simulink model "pwm_analysis"  (R2016a)
settings: Solver=ode4  StartTime=0.0  StopTime=Tfinal  FixedStep=Ts  RelTol=1e-3
undefined symbols (not defined in the file or in its folder): Cdc, delta, deltad, fsw, Lload, ma, phase, Rin, Rload, Ts, Vin, wout
libraries: powerlib x21, powerlib_meascontrol x16
settings Model: Creator=ugurm  LastModifiedBy=mesutto
settings DataIOCC: LimitDataPoints=on  SaveFormat=Array
settings DebuggingCC: UnderspecifiedInitializationDetection=Classic  MergeDetectMultiDrivingBlocksExec=none  SolverPrmCheckMsg=warning  StateNameClashWarn=warning
settings HardwareCC: ProdBitPerPointer=32  ProdLargestAtomicFloat=None  ProdIntDivRoundTo=Undefined  ProdEndianess=Unspecified  ProdWordSize=32  ProdHWDeviceType=32-bit Generic
settings ModelReferenceCC: PropagateSignalLabelsOutOfModel=off
settings ConfigComp: CovModelRefEnable=Off

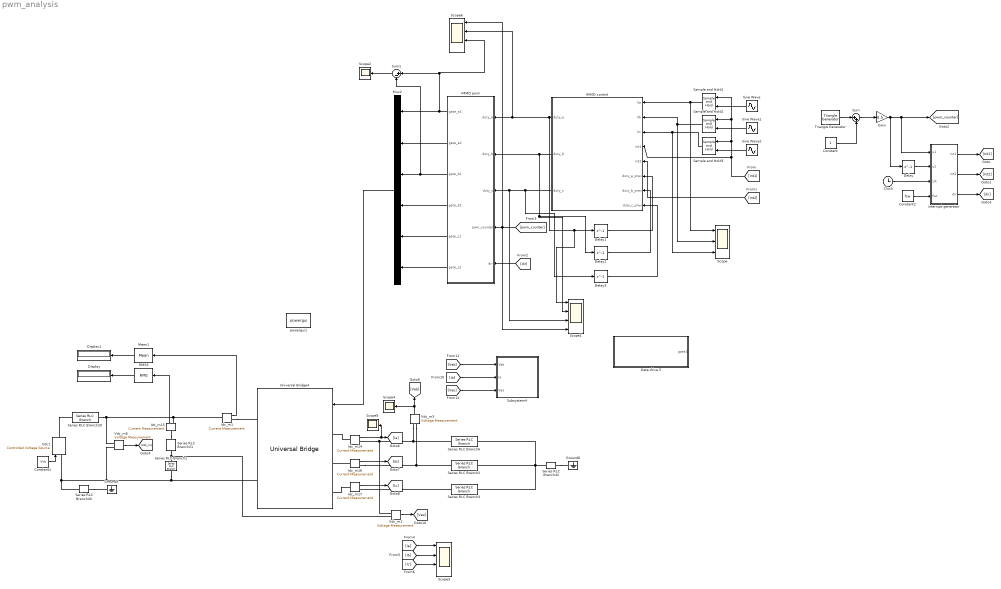
== system pwm_analysis ==
  Clock : Clock
  Constant : Constant
  Constant1 : Constant  Value=Vin
  Constant2 : Constant  Value=fsw
  Delay{,1..3} (4 alike) : Delay  DelayLength=1
  Display : Display
  Display1 : Display
  Gain : Gain  Gain=0.5
  Gate drive 5 : Subsystem
  Ground5 : powerlib/Elements/Ground  LConnTagsString=a
  Ground6 : powerlib/Elements/Ground  LConnTagsString=a
  IMMD control : MATLAB Function  TreatAsAtomicUnit=on
  IMMD pwm : MATLAB Function  TreatAsAtomicUnit=on
  Idc_m{1,14..17} (5 alike) : powerlib/Measurements/Current Measurement  PhasorSimulation=off  OutputType=Complex  PSBequivalent=0
  Mean1 : powerlib_meascontrol/Measurements/Mean  Freq=fout  Vinit=0  Ts=0
  Mux2 : Mux  Inputs=6
  RMS3 : powerlib_meascontrol/Measurements/RMS  TrueRMS=on  Freq=fout  RMSInit=0  Ts=0
  Sample and Hold1 : powerlib_meascontrol/Additional Components/Sample and Hold  ic=0  Ts=0
  Sample and Hold2 : powerlib_meascontrol/Additional Components/Sample and Hold  ic=0  Ts=0
  Sample and Hold3 : powerlib_meascontrol/Additional Components/Sample and Hold  ic=0  Ts=0
  Scope : Scope  NumInputPorts=3
  Scope1 : Scope  NumInputPorts=4
  Scope2 : Scope
  Scope3 : Scope  NumInputPorts=4
  Scope4 : Scope
  Scope5 : Scope
  Scope6 : Scope  NumInputPorts=4
  Series RLC Branch1 : powerlib/Elements/Series RLC Branch  LConnTagsString=__new0  RConnTagsString=__new0  BranchType=C  Resistance=Rload  Inductance=Lload  SetiL0=off  InitialCurrent=0  Capacitance=Cdc*2  Setx0=off  InitialVoltage=0  Measurements=None
  Series RLC Branch2 : powerlib/Elements/Series RLC Branch  LConnTagsString=__new0  RConnTagsString=__new0  BranchType=RL  Resistance=10  Inductance=20e-3  SetiL0=off  InitialCurrent=0  Capacitance=1e-6  Setx0=off  InitialVoltage=0  Measurements=None
  Series RLC Branch20 : powerlib/Elements/Series RLC Branch  LConnTagsString=__new0  RConnTagsString=__new0  BranchType=R  Resistance=Rin  Inductance=Lload  SetiL0=off  InitialCurrent=0  Capacitance=1e-6  Setx0=off  InitialVoltage=0  Measurements=None
  Series RLC Branch21 : powerlib/Elements/Series RLC Branch  LConnTagsString=__new0  RConnTagsString=__new0  BranchType=C  Resistance=Rload  Inductance=Lload  SetiL0=off  InitialCurrent=0  Capacitance=Cdc*2  Setx0=off  InitialVoltage=0  Measurements=None
  Series RLC Branch3 : powerlib/Elements/Series RLC Branch  LConnTagsString=__new0  RConnTagsString=__new0  BranchType=RL  Resistance=10  Inductance=20e-3  SetiL0=off  InitialCurrent=0  Capacitance=1e-6  Setx0=off  InitialVoltage=0  Measurements=None
  Series RLC Branch40 : powerlib/Elements/Series RLC Branch  LConnTagsString=__new0  RConnTagsString=__new0  BranchType=R  Resistance=1e12  Inductance=Lload  SetiL0=off  InitialCurrent=0  Capacitance=1e-6  Setx0=off  InitialVoltage=0  Measurements=None
  Series RLC Branch42 : powerlib/Elements/Series RLC Branch  LConnTagsString=__new0  RConnTagsString=__new0  BranchType=R  Resistance=1e12  Inductance=Lload  SetiL0=off  InitialCurrent=0  Capacitance=1e-6  Setx0=off  InitialVoltage=0  Measurements=None
  Series RLC Branch6 : powerlib/Elements/Series RLC Branch  LConnTagsString=__new0  RConnTagsString=__new0  BranchType=RL  Resistance=10  Inductance=20e-3  SetiL0=off  InitialCurrent=0  Capacitance=1e-6  Setx0=off  InitialVoltage=0  Measurements=None
  Sine Wave : Sin  Amplitude=0.9  Frequency=50*2*pi  SampleTime=0
  Sine Wave1 : Sin  Amplitude=0.9  Frequency=50*2*pi  Phase=2*pi/3  SampleTime=0
  Sine Wave2 : Sin  Amplitude=0.9  Frequency=50*2*pi  Phase=4*pi/3  SampleTime=0
  Subsystem4 : Subsystem
  Sum : Sum  Inputs=|++
  Sum1 : Sum  Inputs=|+-
  Triangle Generator : powerlib_meascontrol/Pulse & Signal Generators/Triangle Generator  Freq=fsw  Phase=0  Ts=0
  Universal Bridge4 : powerlib/Power Electronics/Universal Bridge  Arms=3  SnubberResistance=1e5  SnubberCapacitance=inf  Device=IGBT / Diodes  Ron=1e-6  Lon=0  ForwardVoltages="[  0  0  ]"  ForwardVoltage=0  GTOparameters=[ 10e-6 , 20e-6 ]  IGBTparameters=[0,0]  Measurements=None  Measurements_2=None  converterType=Rectifier
  Vdc1 : powerlib/Electrical Sources/Controlled Voltage Source  Initialize=off  Source_Type=DC  Amplitude=200  Phase=0  Frequency=0  Measurements=None
  Vdc_m1 : powerlib/Measurements/Voltage Measurement  PhasorSimulation=off  OutputType=Complex  PSBequivalent=0
  Vdc_m5 : powerlib/Measurements/Voltage Measurement  PhasorSimulation=off  OutputType=Complex  PSBequivalent=0
  Vdc_m6 : powerlib/Measurements/Voltage Measurement  PhasorSimulation=off  OutputType=Complex  PSBequivalent=0
  interrupt generator : MATLAB Function  TreatAsAtomicUnit=on
  powergui1 : powerlib/powergui  Priority=1  SimulationMode=Discrete  SolverType=Tustin  SampleTime=Ts  frequency=60  SPID=off  DisableSnubberDevices=off  DisableRonSwitches=off  DisableVfSwitches=off  SwTol=0  DisplayEquations=off  Interpol=off  ExternalGateDelay=off  methode=off  Ts=0  FunctionMessages=off  echomessages=off  HookPort=off  EnableUseOfTLC=off  x0status=blocks  frequencyindice=0  Pbase=100e6  ErrMax=1e-4  Iterations=50  UnitsV=kV  UnitsW=MW  buscounter=0  RestoreLinks=warning  ResistiveCurrentMeasurement=off  Frange=[0:2:500]  Ylog=off  Xlog=on  ShowGrid=off  save=off  variable=ZData  structure=ScopeData5  ZoomFFT=off  StartTime=0.02  cycles=2  DisplayStyle=1  fundamental=50  FreqAxis=off  MaxFrequency=50000  frequencyindicesteady=1  RmsSteady=1  display=off
  wires:
  Constant1/1 -> Vdc1/1
  Idc_m15/1 -> RMS3/1
  Vdc_m6/1 -> [Vdc_m]
  RMS3/1 -> Display/1
  Idc_m1/1 -> Mean1/1
  Mean1/1 -> Display1/1
  Triangle Generator/1 -> Sum/1
  Constant/1 -> Sum/2
  Sum/1 -> Gain/1
  Gain/1 -> [pwm_counter], interrupt generator/1(u1), Delay/1
  Delay/1 -> interrupt generator/2(u2)
  Clock/1 -> interrupt generator/3(clk)
  Constant2/1 -> interrupt generator/4(fsw)
  Idc_m14/1 -> Scope5/1, [Ia]
  IMMD pwm/1(gate_a1) -> Scope6/3, Sum1/1, Mux2/1
  IMMD pwm/2(gate_a2) -> Mux2/2
  IMMD pwm/3(gate_b1) -> Sum1/2, Mux2/3
  IMMD pwm/4(gate_b2) -> Mux2/4
  IMMD pwm/5(gate_c1) -> Mux2/5
  IMMD pwm/6(gate_c2) -> Mux2/6
  Sample and Hold3/1 -> Scope/3, IMMD control/3(Vc)
  Sample and Hold2/1 -> Scope/2, IMMD control/2(Vb)
  Sample and Hold1/1 -> Scope/1, IMMD control/1(Va)
  interrupt generator/1(int1) -> [Int1]
  Mux2/1 -> Universal Bridge4/1
  interrupt generator/2(int2) -> [Int2]
  [dir] -> IMMD pwm/5(dir)
  interrupt generator/3(dir) -> [dir]
  [pwm_counter] -> Scope1/4, Scope6/1, IMMD pwm/4(pwm_counter)
  IMMD control/2(duty_b) -> Scope1/2, Delay2/1, IMMD pwm/2(duty_b)
  IMMD control/1(duty_a) -> Scope6/2, IMMD pwm/1(duty_a), Scope1/1, Delay1/1
  [Ia] -> Subsystem4/2(Ia)
  Idc_m16/1 -> [Ib]
  Idc_m17/1 -> [Ic]
  [Vab] -> Subsystem4/1(Vab)
  [Vao] -> Subsystem4/3(Vao)
  Vdc_m5/1 -> [Vab], Scope4/1
  Vdc_m1/1 -> [Vao]
  [Int2] -> IMMD control/5(int2)
  Sine Wave/1 -> Sample and Hold1/1
  Sine Wave1/1 -> Sample and Hold2/1
  Sine Wave2/1 -> Sample and Hold3/1
  [Int1] -> Sample and Hold3/2, Sample and Hold2/2, Sample and Hold1/2, IMMD control/4(int1)
  Delay1/1 -> IMMD control/6(duty_a_prev)
  Delay2/1 -> IMMD control/7(duty_b_prev)
  Delay3/1 -> IMMD control/8(duty_c_prev)
  IMMD control/3(duty_c) -> Delay3/1, Scope1/3, IMMD pwm/3(duty_c)
  Sum1/1 -> Scope2/1
  [Ia] -> Scope3/1
  [Ib] -> Scope3/2
  [Ic] -> Scope3/3
  connections:
  Vdc_m5/LConn1 -- Idc_m14/RConn1 -- Vdc_m1/LConn1 -- Series RLC Branch6/LConn1
  Universal Bridge4/RConn2 -- Vdc_m6/LConn2 -- Vdc1/LConn1 -- Series RLC Branch40/LConn1 -- Series RLC Branch1/RConn1
  Series RLC Branch42/RConn1 -- Ground6/LConn1
  Series RLC Branch40/RConn1 -- Ground5/LConn1
  Idc_m14/LConn1 -- Universal Bridge4/LConn1
  Idc_m15/LConn1 -- Series RLC Branch21/LConn1
  Vdc1/RConn1 -- Series RLC Branch20/LConn1
  Series RLC Branch42/LConn1 -- Series RLC Branch2/RConn1 -- Series RLC Branch3/RConn1 -- Series RLC Branch6/RConn1
  Idc_m16/LConn1 -- Universal Bridge4/LConn2
  Idc_m17/LConn1 -- Universal Bridge4/LConn3
  Series RLC Branch3/LConn1 -- Idc_m17/RConn1
  Idc_m16/RConn1 -- Series RLC Branch2/LConn1 -- Vdc_m5/LConn2
  Idc_m1/RConn1 -- Universal Bridge4/RConn1
  Idc_m1/LConn1 -- Series RLC Branch20/RConn1 -- Vdc_m6/LConn1 -- Idc_m15/RConn1
  Series RLC Branch1/LConn1 -- Vdc_m1/LConn2 -- Series RLC Branch21/RConn1

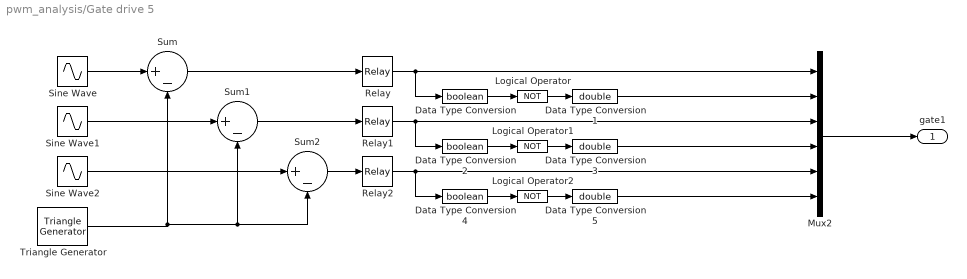
== system pwm_analysis/Gate drive 5 ==
  Data Type Conversion : DataTypeConversion  OutDataTypeStr=boolean
  Data Type Conversion1 : DataTypeConversion  OutDataTypeStr=double
  Data Type Conversion2 : DataTypeConversion  OutDataTypeStr=boolean
  Data Type Conversion3 : DataTypeConversion  OutDataTypeStr=double
  Data Type Conversion4 : DataTypeConversion  OutDataTypeStr=boolean
  Data Type Conversion5 : DataTypeConversion  OutDataTypeStr=double
  Logical Operator : Logic  Operator=NOT  AllPortsSameDT=off  OutDataTypeStr=boolean
  Logical Operator1 : Logic  Operator=NOT  AllPortsSameDT=off  OutDataTypeStr=boolean
  Logical Operator2 : Logic  Operator=NOT  AllPortsSameDT=off  OutDataTypeStr=boolean
  Mux2 : Mux  Inputs=6
  Relay : Relay
  Relay1 : Relay
  Relay2 : Relay
  Sine Wave : Sin  Amplitude=ma  Frequency=wout  Phase=delta  SampleTime=0
  Sine Wave1 : Sin  Amplitude=ma  Frequency=wout  Phase=-2*pi/3+delta  SampleTime=0
  Sine Wave2 : Sin  Amplitude=ma  Frequency=wout  Phase=2*pi/3+delta  SampleTime=0
  Sum : Sum  Inputs=|+-
  Sum1 : Sum  Inputs=|+-
  Sum2 : Sum  Inputs=|+-
  Triangle Generator : powerlib_meascontrol/Pulse & Signal Generators/Triangle Generator  Freq=fsw  Phase=phase(1)  Ts=Ts
  gate1 : Outport
  wires:
  Sine Wave/1 -> Sum/1
  Triangle Generator/1 -> Sum1/2, Sum2/2, Sum/2
  Sine Wave1/1 -> Sum1/1
  Sine Wave2/1 -> Sum2/1
  Sum/1 -> Relay/1
  Sum1/1 -> Relay1/1
  Sum2/1 -> Relay2/1
  Data Type Conversion/1 -> Logical Operator/1
  Relay/1 -> Data Type Conversion/1, Mux2/1
  Logical Operator/1 -> Data Type Conversion1/1
  Data Type Conversion1/1 -> Mux2/2
  Data Type Conversion2/1 -> Logical Operator1/1
  Relay1/1 -> Data Type Conversion2/1, Mux2/3
  Logical Operator1/1 -> Data Type Conversion3/1
  Data Type Conversion3/1 -> Mux2/4
  Data Type Conversion4/1 -> Logical Operator2/1
  Relay2/1 -> Data Type Conversion4/1, Mux2/5
  Logical Operator2/1 -> Data Type Conversion5/1
  Data Type Conversion5/1 -> Mux2/6
  Mux2/1 -> gate1/1

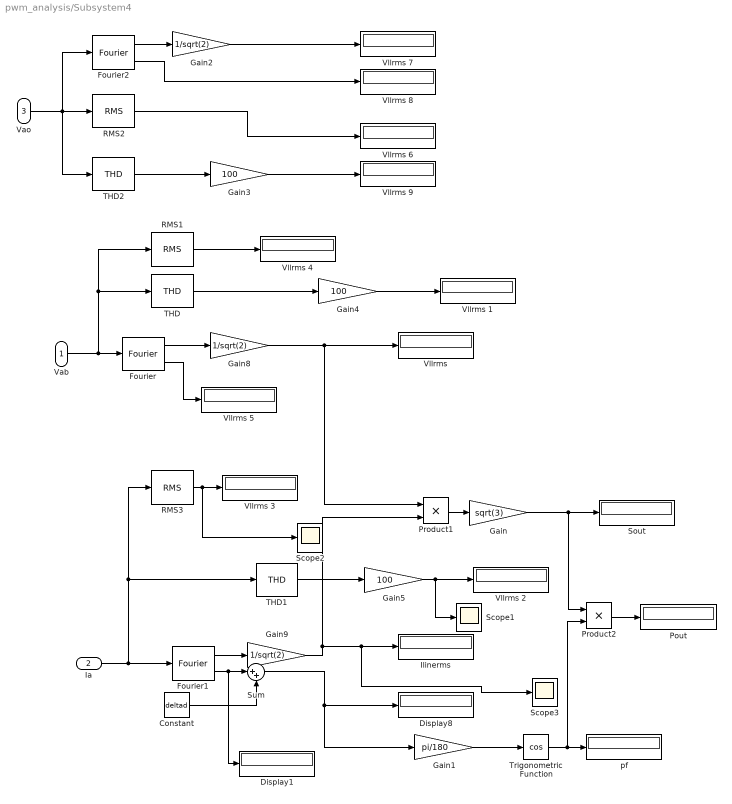
== system pwm_analysis/Subsystem4 ==
  Vab : Inport
  Ia : Inport  Port=2
  Vao : Inport  Port=3
  Constant : Constant  Value=deltad
  Display1 : Display
  Display8 : Display
  Fourier : powerlib_meascontrol/Measurements/Fourier  Freq=fout  n=1  InInit=[0, 0]  Ts=Ts
  Fourier1 : powerlib_meascontrol/Measurements/Fourier  Freq=fout  n=1  InInit=[0, 0]  Ts=Ts
  Fourier2 : powerlib_meascontrol/Measurements/Fourier  Freq=fout  n=1  InInit=[0, 0]  Ts=Ts
  Gain : Gain  Gain=sqrt(3)
  Gain1 : Gain  Gain=pi/180
  Gain2 : Gain  Gain=1/sqrt(2)
  Gain3 : Gain  Gain=100
  Gain4 : Gain  Gain=100
  Gain5 : Gain  Gain=100
  Gain8 : Gain  Gain=1/sqrt(2)
  Gain9 : Gain  Gain=1/sqrt(2)
  "Ilinerms " : Display
  Pout : Display
  Product1 : Product
  Product2 : Product
  RMS1 : powerlib_meascontrol/Measurements/RMS  TrueRMS=on  Freq=fout  RMSInit=0  Ts=0
  RMS2 : powerlib_meascontrol/Measurements/RMS  TrueRMS=on  Freq=fout  RMSInit=0  Ts=0
  RMS3 : powerlib_meascontrol/Measurements/RMS  TrueRMS=on  Freq=fout  RMSInit=0  Ts=0
  Scope1 : Scope
  Scope2 : Scope
  Scope3 : Scope
  Sout : Display
      settings: Format=short_e
  Sum : Sum  Inputs=|++
  THD : powerlib_meascontrol/Measurements/THD  Freq=fout  Ts=0
  THD1 : powerlib_meascontrol/Measurements/THD  Freq=fout  Ts=0
  THD2 : powerlib_meascontrol/Measurements/THD  Freq=fout  Ts=0
  Trigonometric Function : Trigonometry  Operator=cos
  Vllrms {,1..9} (10 alike) : Display
  pf : Display
  wires:
  Gain8/1 -> Product1/1, "Vllrms "/1
  Gain9/1 -> Scope3/1, "Ilinerms "/1, Product1/2
  Ia/1 -> RMS3/1, THD1/1, Fourier1/1
  Fourier1/1 -> Gain9/1
  Vab/1 -> RMS1/1, THD/1, Fourier/1
  Fourier/1 -> Gain8/1
  Product1/1 -> Gain/1
  Gain/1 -> Product2/1, Sout/1
  Sum/1 -> Gain1/1, Display8/1
  Trigonometric Function/1 -> Product2/2, pf/1
  Gain1/1 -> Trigonometric Function/1
  Product2/1 -> Pout/1
  Fourier/2 -> Vllrms 5/1
  THD/1 -> Gain4/1
  THD1/1 -> Gain5/1
  Constant/1 -> Sum/2
  RMS3/1 -> Scope2/1, Vllrms 3/1
  RMS1/1 -> Vllrms 4/1
  Fourier1/2 -> Display1/1, Sum/1
  Vao/1 -> THD2/1, Fourier2/1, RMS2/1
  RMS2/1 -> Vllrms 6/1
  Fourier2/1 -> Gain2/1
  Fourier2/2 -> Vllrms 8/1
  Gain2/1 -> Vllrms 7/1
  THD2/1 -> Gain3/1
  Gain3/1 -> Vllrms 9/1
  Gain4/1 -> Vllrms 1/1
  Gain5/1 -> Scope1/1, Vllrms 2/1

== matlab function pwm_analysis/IMMD control ==
  data: Va input; duty_a output; Vb input; Vc input; duty_b output; duty_c output; int1 input; int2 input; duty_a_prev input; duty_b_prev input; duty_c_prev input
function [duty_a,duty_b,duty_c] = fcn(Va,Vb,Vc,int1,int2,...
    duty_a_prev,duty_b_prev,duty_c_prev)

if (int1 == 1) % interrupt on zero event  
    duty_a = (Va+1)/2;
    duty_b = (Vb+1)/2;
    duty_c = (Vc+1)/2;
    
else
    duty_a = duty_a_prev; %//
    duty_b = duty_b_prev; %//
    duty_c = duty_c_prev; %//
    
end;

% if (int2 == 1) % interrupt on prd event
%     duty_a = duty_a_temp;
%     duty_b = duty_b_temp;
%     duty_c = duty_c_temp;
% else
%     duty_a = 1; %//
%     duty_b = 1; %//
%     duty_c = 1; %//
% end;

== matlab function pwm_analysis/interrupt generator ==
  data: u1 input; int1 output; u2 input; clk input; int2 output; dir output; fsw input
function [int1,int2,dir] = fcn(u1,u2,clk,fsw)

if (rem(clk,1/fsw) == 0)
    int1 = 1; % interrupt on zero
    dir = 0;
else
    int1 = 0;
    if (u1 > u2)
        dir = 1; % up
    else
        dir = 0; % down
    end;
end;

if (rem(clk*2,1/fsw) == 0 && rem(clk,1/fsw) ~= 0)
    int2 = 1; % interrupt on period
else
    int2 = 0;
end;

== matlab function pwm_analysis/IMMD pwm ==
  data: duty_a input; gate_a1 output; duty_b input; duty_c input; gate_a2 output; gate_b1 output; gate_b2 output; gate_c1 output; gate_c2 output; pwm_counter input; dir input
function [gate_a1,gate_a2,gate_b1,gate_b2,gate_c1,gate_c2] = fcn(duty_a,duty_b,duty_c,pwm_counter,dir)

%if (dir == 1)
    if (duty_a > pwm_counter)
        gate_a1 = 1;
        gate_a2 = 0;
    else
        gate_a1 = 0;
        gate_a2 = 1;
    end;
    if (duty_b > pwm_counter)
        gate_b1 = 1;
        gate_b2 = 0;
    else
        gate_b1 = 0;
        gate_b2 = 1;
    end;
    if (duty_c > pwm_counter)
        gate_c1 = 1;
        gate_c2 = 0;
    else
        gate_c1 = 0;
        gate_c2 = 1;
    end;

%     if (duty_a > pwm_counter)
%         gate_a1 = 0;
%         gate_a2 = 1;
%     else
%         gate_a1 = 1;
%         gate_a2 = 0;
%     end;
%     if (duty_b > pwm_counter)
%         gate_b1 = 0;
%         gate_b2 = 1;
%     else
%         gate_b1 = 1;
%         gate_b2 = 0;
%     end;
%     if (duty_c > pwm_counter)
%         gate_c1 = 0;
%         gate_c2 = 1;
%     else
%         gate_c1 = 1;
%         gate_c2 = 0;
%     end;
    
%else
    

%end;
